simulink model "IMU_int"  (R2023b)
settings: Solver=ode4  StartTime=0.0  StopTime=10000  FixedStep=clock.sampleTime.value  RelTol=1e-3
undefined symbols (not defined in the file or in its folder): DiscIntNeverNeededParam, IMU, MainSpacecraft, Propagation
libraries: sharedtransform x4, dyn_lib x3, nav_lib x3, vrlib x2
settings Model: DataDictionary=SimulationDict.sldd  EnableAccessToBaseWorkspace=off  Creator=brent  LastModifiedBy=brent

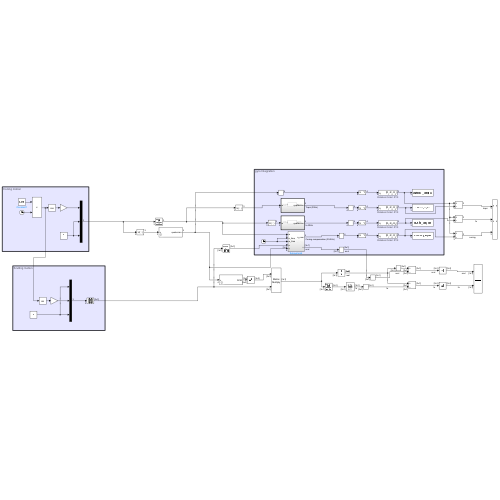
[thumbnail: Simulink's stored preview of the top-level diagram]
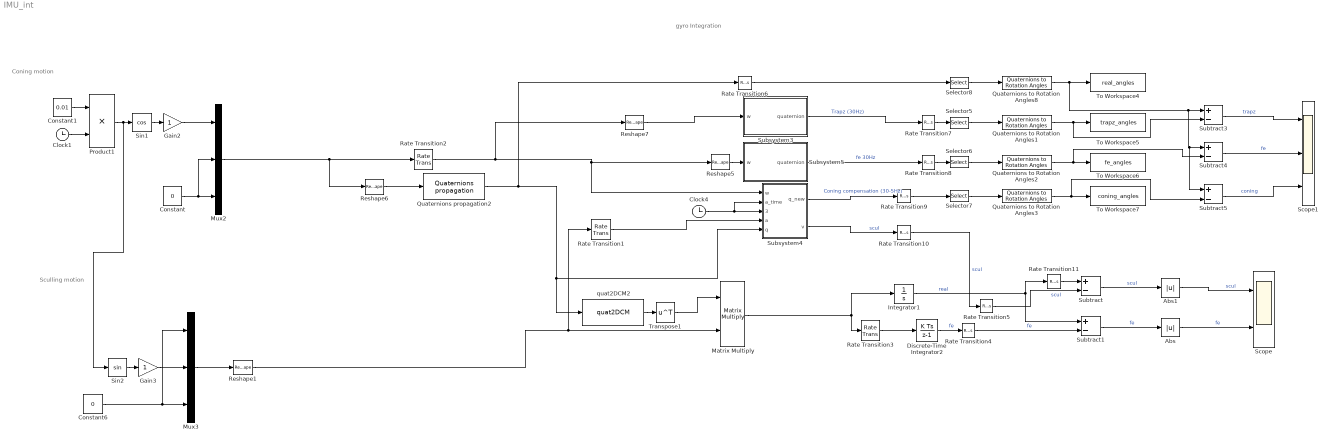
== system IMU_int ==
  note: Coning motion
  note: Sculling motion
  note: gyro Integration
  Abs : Abs  SaturateOnIntegerOverflow=off
  Abs1 : Abs  SaturateOnIntegerOverflow=off
  Clock1 : Clock
  Clock4 : Clock
  Constant : Constant  Value=0
  Constant1 : Constant  Value=0.01
  Constant6 : Constant  Value=0
  Discrete-Time Integrator2 : DiscreteIntegrator  SampleTime=-1  ICPrevOutput=DiscIntNeverNeededParam  ICPrevScaledInput=DiscIntNeverNeededParam
  Gain2 : Gain
  Gain3 : Gain
  Integrator1 : Integrator  InitialCondition=[0;0;0]
  Matrix Multiply : Product  Multiplication=Matrix(*)
  Mux2 : Mux  Inputs=3
  Mux3 : Mux  Inputs=3
  Product1 : Product
  Quaternions propagation2 : dyn_lib/Quaternions propagation  q0=MainSpacecraft.q0.value
      settings: SourceProductName=Dynamics library
  Quaternions to Rotation Angles{1..3,8} (4 alike) : sharedtransform/Quaternions to Rotation Angles  rotationOrder=ZYX  aMode=aMode
  Rate Transition1 : RateTransition  InitialCondition=[0;0;0]  OutPortSampleTime=1/30
  Rate Transition10 : RateTransition  InitialCondition=[0;0;0]  OutPortSampleTime=1/Propagation.lf.value
  Rate Transition11 : RateTransition  OutPortSampleTime=0.2
  Rate Transition2 : RateTransition  InitialCondition=[0;0;0]  OutPortSampleTime=1/30
  Rate Transition3 : RateTransition  InitialCondition=[0;0;0]  OutPortSampleTime=1/30
  Rate Transition4 : RateTransition  OutPortSampleTime=0.2
  Rate Transition5 : RateTransition  OutPortSampleTime=0.2
  Rate Transition{6..9} (4 alike) : RateTransition  InitialCondition=MainSpacecraft.q0.value  OutPortSampleTime=1/Propagation.lf.value
  Reshape1 : Reshape  OutputDimensionality=Column vector (2-D)
  Reshape5 : Reshape
  Reshape6 : Reshape
  Reshape7 : Reshape
  Scope : Scope  NumInputPorts=2
  Scope1 : Scope  NumInputPorts=3
  Selector{5..8} (4 alike) : Selector  InputPortWidth=4  IndexOptions=Index vector (dialog)  Indices=[2 3 4 1]  OutputSizes=1
  Sin1 : Trigonometry  Operator=cos
  Sin2 : Trigonometry
  Subsystem3 : Subsystem  TreatAsAtomicUnit=on  SystemSampleTime=1/30
  Subsystem4 : Subsystem  SystemSampleTime=1/30
  Subsystem5 : Subsystem  TreatAsAtomicUnit=on  SystemSampleTime=IMU.gyroscope.sampleTime.value
  Subtract{,1,3..5} (5 alike) : Sum  Inputs=+-
  To Workspace4 : ToWorkspace  VariableName=real_angles  SaveFormat=Timeseries  SampleTime=-1
  To Workspace5 : ToWorkspace  VariableName=trapz_angles  SaveFormat=Timeseries  SampleTime=-1
  To Workspace6 : ToWorkspace  VariableName=fe_angles  SaveFormat=Timeseries  SampleTime=-1
  To Workspace7 : ToWorkspace  VariableName=coning_angles  SaveFormat=Timeseries  SampleTime=-1
  Transpose1 : Math  Operator=transpose
  quat2DCM2 : dyn_lib/quat2DCM
      settings: SourceProductName=Dynamics library
  wires:
  Reshape7/1 -> Subsystem3/1(w)
  Rate Transition10/1 -> Rate Transition5/1  "scul"
  Reshape6/1 -> Quaternions propagation2/1
  Reshape5/1 -> Subsystem5/1(w)
  Sin2/1 -> Gain3/1
  Selector6/1 -> Quaternions to Rotation Angles2/1
  Rate Transition7/1 -> Selector5/1
  Selector5/1 -> Quaternions to Rotation Angles1/1
  Subsystem4/2(v) -> Rate Transition10/1  "scul"
  Rate Transition9/1 -> Selector7/1
  Quaternions to Rotation Angles8/1 -> Subtract5/1, Subtract4/1, Subtract3/1, To Workspace4/1
  Selector8/1 -> Quaternions to Rotation Angles8/1
  Rate Transition8/1 -> Selector6/1
  Quaternions to Rotation Angles1/1 -> Subtract3/2, To Workspace5/1
  Quaternions to Rotation Angles2/1 -> Subtract4/2, To Workspace6/1
  Quaternions to Rotation Angles3/1 -> Subtract5/2, To Workspace7/1
  Subsystem3/1(quaternion) -> Rate Transition7/1  "Trapz (30Hz)"
  Rate Transition6/1 -> Selector8/1
  Selector7/1 -> Quaternions to Rotation Angles3/1
  Clock4/1 -> Subsystem4/2(a_time), Subsystem4/3(w_time)
  Subsystem4/1(q_new) -> Rate Transition9/1  "Coning compensation (30-5Hz)"
  Gain2/1 -> Mux2/1
  Constant6/1 -> Mux3/1, Mux3/3
  Product1/1 -> Sin2/1, Sin1/1
  quat2DCM2/1 -> Transpose1/1
  Transpose1/1 -> Matrix Multiply/1
  Mux3/1 -> Reshape1/1
  Matrix Multiply/1 -> Integrator1/1, Rate Transition3/1
  Subtract3/1 -> Scope1/1  "trapz"
  Subtract4/1 -> Scope1/2  "fe"
  Subtract5/1 -> Scope1/3  "coning"
  Subsystem5/1(quaternion) -> Rate Transition8/1  "fe 30Hz"
  Gain3/1 -> Mux3/2
  Integrator1/1 -> Rate Transition11/1, Subtract1/1  "real"
  Discrete-Time Integrator2/1 -> Rate Transition4/1  "fe"
  Reshape1/1 -> Rate Transition1/1, Matrix Multiply/2
  Mux2/1 -> Reshape6/1, Rate Transition2/1
  Rate Transition2/1 -> Subsystem4/1(w), Reshape5/1, Reshape7/1
  Rate Transition1/1 -> Subsystem4/4(a)
  Rate Transition3/1 -> Discrete-Time Integrator2/1
  Constant/1 -> Mux2/2, Mux2/3
  Constant1/1 -> Product1/1
  Clock1/1 -> Product1/2
  Sin1/1 -> Gain2/1
  Rate Transition4/1 -> Subtract1/2  "fe"
  Rate Transition5/1 -> Subtract/2  "scul"
  Quaternions propagation2/1 -> Rate Transition6/1, Subsystem4/5(q), quat2DCM2/1
  Rate Transition11/1 -> Subtract/1
  Subtract/1 -> Abs1/1  "scul"
  Subtract1/1 -> Abs/1  "fe"
  Abs/1 -> Scope/2  "fe"
  Abs1/1 -> Scope/1  "scul"

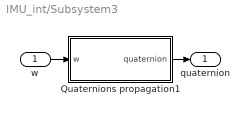
== system IMU_int/Subsystem3 ==
  w : Inport
  Quaternions propagation1 : Subsystem  AncestorBlock=dyn_lib/Quaternions propagation  mask{q0=MainSpacecraft.q0.value}
      mask prompts: q0 "Initial attitude quaternion"
      mask DialogControl DescGroupVar Prompt: Quaternion propagation
  quaternion : Outport
  wires:
  w/1 -> Quaternions propagation1/1(w)
  Quaternions propagation1/1(quaternion) -> quaternion/1

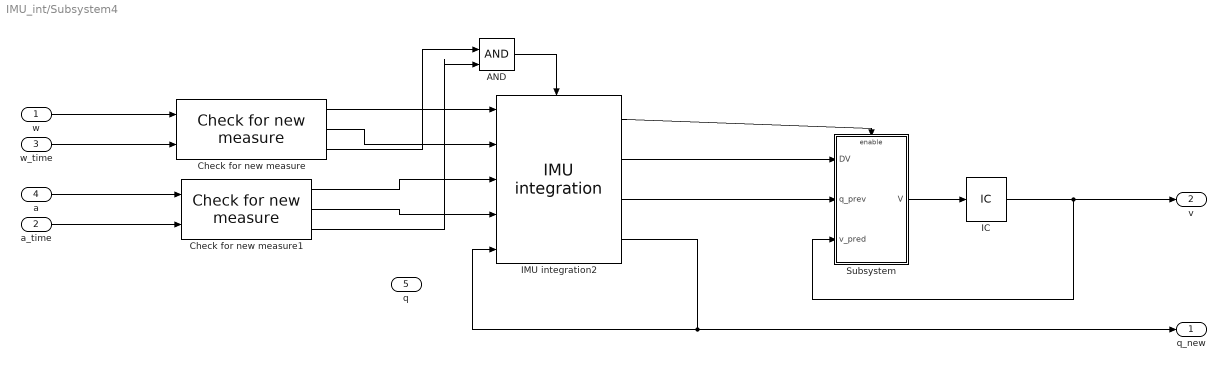
== system IMU_int/Subsystem4 ==
  w : Inport
  a_time : Inport  Port=2
  w_time : Inport  Port=3
  a : Inport  Port=4
  q : Inport  Port=5
  AND : Logic  IconShape=distinctive  AllPortsSameDT=off  OutDataTypeStr=boolean
  Check for new measure : nav_lib/Check for new measure  Ts=1/30
      settings: SourceProductName=Navigation library
  Check for new measure1 : nav_lib/Check for new measure  Ts=1/30
      settings: SourceProductName=Navigation library
  IC : InitialCondition  Value=[0;0;0]
  IMU integration2 : nav_lib/IMU integration  HF=30  LF=5  q0=MainSpacecraft.q0.value
      settings: SourceProductName=Navigation library
  Subsystem : Subsystem
  q_new : Outport
  v : Outport  Port=2
  wires:
  IMU integration2/4 -> IMU integration2/5, q_new/1
  IMU integration2/2 -> Subsystem/1(DV)
  Check for new measure/1 -> IMU integration2/1
  AND/1 -> IMU integration2/Enable
  IMU integration2/1 -> Subsystem/Enable
  Check for new measure1/1 -> IMU integration2/3
  Check for new measure/2 -> IMU integration2/2
  Subsystem/1(V) -> IC/1
  IC/1 -> Subsystem/3(v_pred), v/1
  Check for new measure/3 -> AND/1
  Check for new measure1/3 -> AND/2
  w/1 -> Check for new measure/1
  w_time/1 -> Check for new measure/2
  a_time/1 -> Check for new measure1/2
  a/1 -> Check for new measure1/1
  Check for new measure1/2 -> IMU integration2/4
  IMU integration2/3 -> Subsystem/2(q_prev)

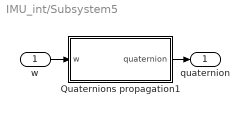
== system IMU_int/Subsystem5 ==
  w : Inport
  Quaternions propagation1 : Subsystem  AncestorBlock=dyn_lib/Quaternions propagation  mask{q0=MainSpacecraft.q0.value}
      mask prompts: q0 "Initial attitude quaternion"
      mask DialogControl DescGroupVar Prompt: Quaternion propagation
  quaternion : Outport
  wires:
  Quaternions propagation1/1(quaternion) -> quaternion/1
  w/1 -> Quaternions propagation1/1(w)

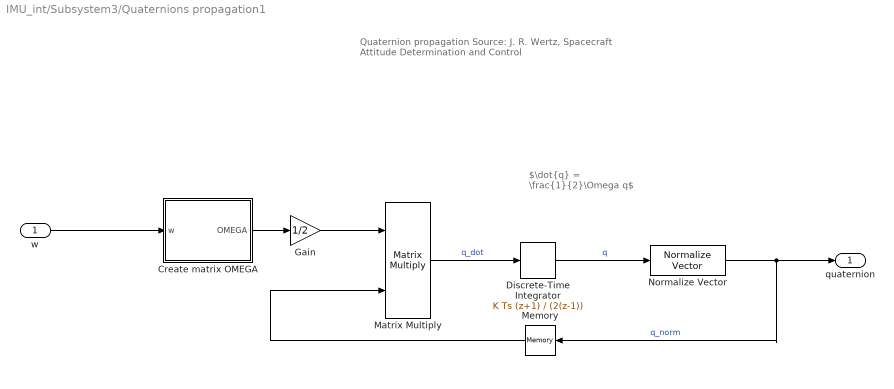
== system IMU_int/Subsystem3/Quaternions propagation1 ==
  note: $\dot{q} = \frac{1}{2}\Omega q$
  note: Quaternion propagation
      |
      | Source:
      | J. R. Wertz, Spacecraft Attitude Determination and Control
  w : Inport
  Create matrix OMEGA : Subsystem
  Discrete-Time Integrator : DiscreteIntegrator  IntegratorMethod=Integration: Trapezoidal  InitialCondition=q0  SampleTime=-1  ICPrevOutput=DiscIntNeverNeededParam  ICPrevScaledInput=DiscIntNeverNeededParam
  Gain : Gain  Gain=1/2  SaturateOnIntegerOverflow=on  OutDataTypeStr=Inherit: Same as input  ParamDataTypeStr=Inherit: Same as input
  Matrix Multiply : Product  Multiplication=Matrix(*)
  Memory : Memory  InitialCondition=q0  InheritSampleTime=on
  Normalize Vector : vrlib/Utilities/Normalize Vector  maxzero=0
  quaternion : Outport
  wires:
  w/1 -> Create matrix OMEGA/1(w)
  Matrix Multiply/1 -> Discrete-Time Integrator/1  "q_dot"
  Normalize Vector/1 -> quaternion/1, Memory/1  "q_norm"
  Discrete-Time Integrator/1 -> Normalize Vector/1  "q"
  Create matrix OMEGA/1(OMEGA) -> Gain/1
  Gain/1 -> Matrix Multiply/1
  Memory/1 -> Matrix Multiply/2

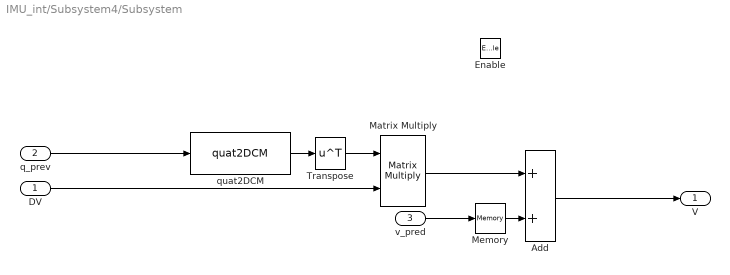
== system IMU_int/Subsystem4/Subsystem ==
  DV : Inport
  q_prev : Inport  Port=2
  v_pred : Inport  Port=3
  Enable : EnablePort
  Add : Sum
  Matrix Multiply : Product  Multiplication=Matrix(*)
  Memory : Memory  InitialCondition=[0;0;0]  InheritSampleTime=on
  Transpose : Math  Operator=transpose
  quat2DCM : dyn_lib/quat2DCM
      settings: SourceProductName=Dynamics library
  V : Outport
  wires:
  Add/1 -> V/1
  v_pred/1 -> Memory/1
  Memory/1 -> Add/2
  DV/1 -> Matrix Multiply/2
  quat2DCM/1 -> Transpose/1
  Transpose/1 -> Matrix Multiply/1
  q_prev/1 -> quat2DCM/1
  Matrix Multiply/1 -> Add/1

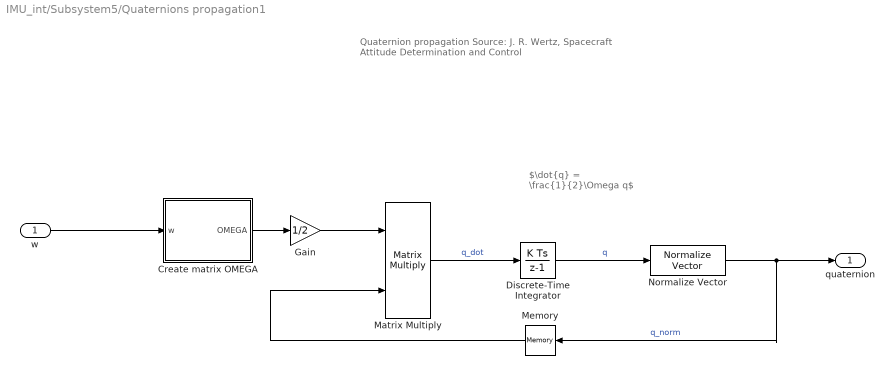
== system IMU_int/Subsystem5/Quaternions propagation1 ==
  note: Quaternion propagation
      |
      | Source:
      | J. R. Wertz, Spacecraft Attitude Determination and Control
  note: $\dot{q} = \frac{1}{2}\Omega q$
  w : Inport
  Create matrix OMEGA : Subsystem
  Discrete-Time Integrator : DiscreteIntegrator  InitialCondition=q0  SampleTime=-1  ICPrevOutput=DiscIntNeverNeededParam  ICPrevScaledInput=DiscIntNeverNeededParam
  Gain : Gain  Gain=1/2  SaturateOnIntegerOverflow=on  OutDataTypeStr=Inherit: Same as input  ParamDataTypeStr=Inherit: Same as input
  Matrix Multiply : Product  Multiplication=Matrix(*)
  Memory : Memory  InitialCondition=q0  InheritSampleTime=on
  Normalize Vector : vrlib/Utilities/Normalize Vector  maxzero=0
  quaternion : Outport
  wires:
  Memory/1 -> Matrix Multiply/2
  Gain/1 -> Matrix Multiply/1
  Create matrix OMEGA/1(OMEGA) -> Gain/1
  Discrete-Time Integrator/1 -> Normalize Vector/1  "q"
  Normalize Vector/1 -> Memory/1, quaternion/1  "q_norm"
  Matrix Multiply/1 -> Discrete-Time Integrator/1  "q_dot"
  w/1 -> Create matrix OMEGA/1(w)

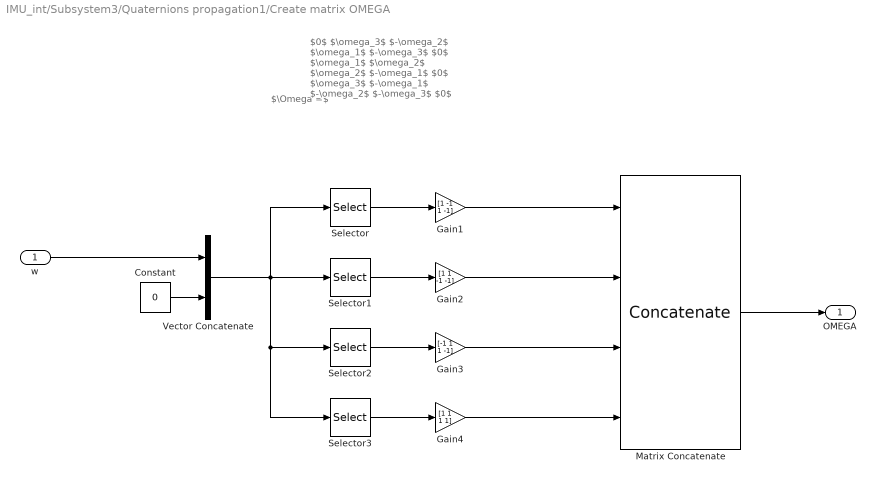
== system IMU_int/Subsystem3/Quaternions propagation1/Create matrix OMEGA ==
  note: $\Omega =$
  note: $0$
      | $\omega_3$
      | $-\omega_2$
      | $\omega_1$
      |
      | $-\omega_3$
      | $0$
      | $\omega_1$
      | $\omega_2$
      |
      | $\omega_2$
      | $-\omega_1$
      | $0$
      | $\omega_3$
      |
      | $-\omega_1$
      | $-\omega_2$
      | $-\omega_3$
      | $0$
  w : Inport
  Constant : Constant  Value=0
  Gain1 : Gain  Gain=[1 -1 1 -1]
  Gain2 : Gain  Gain=[1 1 -1 -1]
  Gain3 : Gain  Gain=[-1 1 1 -1]
  Gain4 : Gain  Gain=[1 1 1 1]
  Matrix Concatenate : Concatenate  NumInputs=4  Mode=Multidimensional array  ConcatenateDimension=2
  Selector : Selector  InputPortWidth=4  IndexOptions=Index vector (dialog)  Indices=[4 3 2 1]  OutputSizes=1
  Selector1 : Selector  InputPortWidth=4  IndexOptions=Index vector (dialog)  Indices=[3 4 1 2]  OutputSizes=1
  Selector2 : Selector  InputPortWidth=4  IndexOptions=Index vector (dialog)  Indices=[2 1 4 3]  OutputSizes=1
  Selector3 : Selector  InputPortWidth=4  IndexOptions=Index vector (dialog)  Indices=[1 2 3 4]  OutputSizes=1
  Vector Concatenate : Concatenate
  OMEGA : Outport
  wires:
  Selector/1 -> Gain1/1
  Selector2/1 -> Gain3/1
  Selector3/1 -> Gain4/1
  Vector Concatenate/1 -> Selector/1, Selector1/1, Selector3/1, Selector2/1
  Constant/1 -> Vector Concatenate/2
  Selector1/1 -> Gain2/1
  Matrix Concatenate/1 -> OMEGA/1
  w/1 -> Vector Concatenate/1
  Gain1/1 -> Matrix Concatenate/1
  Gain2/1 -> Matrix Concatenate/2
  Gain3/1 -> Matrix Concatenate/3
  Gain4/1 -> Matrix Concatenate/4

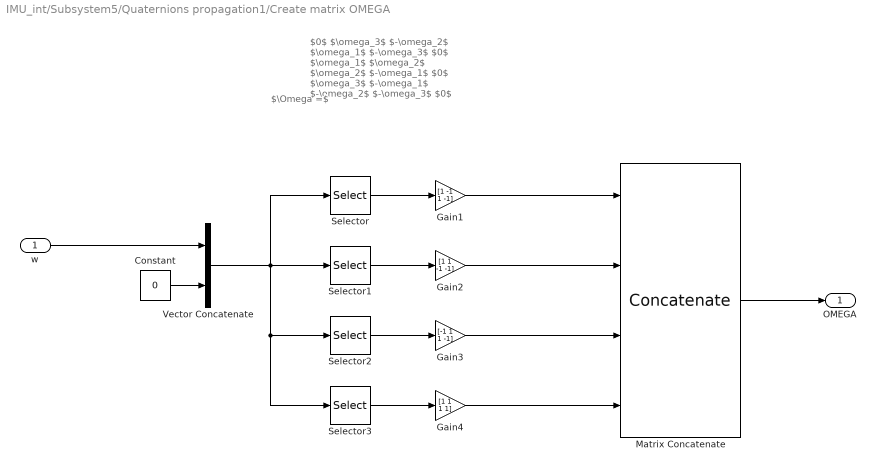
== system IMU_int/Subsystem5/Quaternions propagation1/Create matrix OMEGA ==
  note: $0$
      | $\omega_3$
      | $-\omega_2$
      | $\omega_1$
      |
      | $-\omega_3$
      | $0$
      | $\omega_1$
      | $\omega_2$
      |
      | $\omega_2$
      | $-\omega_1$
      | $0$
      | $\omega_3$
      |
      | $-\omega_1$
      | $-\omega_2$
      | $-\omega_3$
      | $0$
  note: $\Omega =$
  w : Inport
  Constant : Constant  Value=0
  Gain1 : Gain  Gain=[1 -1 1 -1]
  Gain2 : Gain  Gain=[1 1 -1 -1]
  Gain3 : Gain  Gain=[-1 1 1 -1]
  Gain4 : Gain  Gain=[1 1 1 1]
  Matrix Concatenate : Concatenate  NumInputs=4  Mode=Multidimensional array  ConcatenateDimension=2
  Selector : Selector  InputPortWidth=4  IndexOptions=Index vector (dialog)  Indices=[4 3 2 1]  OutputSizes=1
  Selector1 : Selector  InputPortWidth=4  IndexOptions=Index vector (dialog)  Indices=[3 4 1 2]  OutputSizes=1
  Selector2 : Selector  InputPortWidth=4  IndexOptions=Index vector (dialog)  Indices=[2 1 4 3]  OutputSizes=1
  Selector3 : Selector  InputPortWidth=4  IndexOptions=Index vector (dialog)  Indices=[1 2 3 4]  OutputSizes=1
  Vector Concatenate : Concatenate
  OMEGA : Outport
  wires:
  Gain4/1 -> Matrix Concatenate/4
  Gain3/1 -> Matrix Concatenate/3
  Gain2/1 -> Matrix Concatenate/2
  Gain1/1 -> Matrix Concatenate/1
  w/1 -> Vector Concatenate/1
  Matrix Concatenate/1 -> OMEGA/1
  Selector1/1 -> Gain2/1
  Constant/1 -> Vector Concatenate/2
  Vector Concatenate/1 -> Selector2/1, Selector3/1, Selector1/1, Selector/1
  Selector3/1 -> Gain4/1
  Selector2/1 -> Gain3/1
  Selector/1 -> Gain1/1
